simulink model "VissimConnector"  (R2021a)
settings: Solver=FixedStepDiscrete  StartTime=0.0  StopTime=Inf  RelTol=1e-3
libraries: drivingscenarioandsensors x2
settings Model: EnablePacing=on  PacingRate=0.200000  Creator=hichikaw  LastModifiedBy=itik
settings SolverCC: AlgebraicLoopSolver=TrustRegion
settings DataIOCC: SaveOutput=off  SignalLogging=off  DSMLogging=off  SaveTime=off  ReturnWorkspaceOutputs=off
settings OptimizationCC: DefaultParameterBehavior=Inlined  UseDivisionForNetSlopeComputation=on  GainParamInheritBuiltInType=on  UseFloatMulNetSlope=on  InlineInvariantSignals=on  PassReuseOutputArgsAs=Individual arguments  ZeroExternalMemoryAtStartup=off  ZeroInternalMemoryAtStartup=off  NoFixptDivByZeroProtection=on  EfficientFloat2IntCast=on  LifeSpan=1  OptimizeBlockOrder=speed  DifferentSizesBufferReuse=on  EfficientTunableParamExpr=on
settings DebuggingCC: ParameterTunabilityLossMsg=error  SFMachineParentedDataDiag=warning
settings HardwareCC: ProdLongLongMode=on
settings SFSimCC: MATLABDynamicMemAlloc=off
settings RTWCC: SystemTargetFile=ert.tlc  TemplateMakefile=ert_default_tmf
settings CodeAppCC: ForceParamTrailComments=on  IgnoreCustomStorageClasses=off  OperatorAnnotations=on  SimulinkDataObjDesc=on  SFDataObjDesc=on  CustomSymbolStrGlobalVar=rt$N$M  CustomSymbolStrType=$N$M  CustomSymbolStrFcn=$N$M$F  CustomSymbolStrMacro=$N$M  InsertBlockDesc=on
settings ERTTargetCC: TargetLangStandard=C99 (ISO)  GenerateSampleERTMain=on  IncludeMdlTerminateFcn=off  CombineSignalStateStructs=on  SuppressErrorStatus=on  SupportAbsoluteTime=off  SupportComplex=off  InlinedParameterPlacement=NonHierarchical  ERTCustomFileTemplate=example_file_process.tlc  ERTFilePackagingFormat=CompactWithDataFile

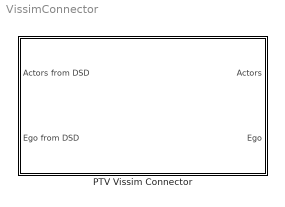
== system VissimConnector ==
  PTV Vissim Connector : Subsystem  mask{msk_strFilename=MyVIssimScenario.inpx, msk_dFrequency=10, msk_dRadius=-1, msk_dMaxNumActors=50, msk_strVissimConnectorDLLFile=./dll/VissimConnectorDLL.dll, msk_strInterfaceDLLFile=./dll/VissimInterfaceInterface.dll, msk_strVissimDLLFile=C:\Program Files\PTV Vision\PTV Vissim 2021\API\DrivingSimulator_DLL\bin\VS2013\x64\DrivingSimulatorProxy.dll}
      mask prompts: msk_strFilename "Vissim file name (*.inpx)"; msk_dFrequency "Vissim simulation frequency (Hz)"; msk_dRadius "Radius to detect actors (m)"; msk_dMaxNumActors "Maximum number of actors"; msk_strVissimConnectorDLLFile "Path to Vissim Connnector DLL<br/>(VissimConnectorDLL.dll)"; msk_strInterfaceDLLFile "Path to Vissim Interface DLL file<br/>(VissimInterfaceInterface.dll)"; msk_strVissimDLLFile "Path to Driving Simulator Proxy DLL<br/>(DrivingSimulatorProxy.dll)"
      mask DialogControl DescTextVar Prompt: Connect to PTV Vissim and interact traffic flow.
      mask DialogControl tab1 Prompt: Parameters
      mask DialogControl msk_btnSelectFile1 Prompt: Select file...
      mask DialogControl msk_btnSelectFile1 Callback:
      | filename = callbackFilenameFromDialog(...
      |     {...
      |         '*.inpx','Vissim (*.inpx)'
      |         '*.*','All (*.*)'}, ...
      |     gcb,'msk_strFilename');
      mask DialogControl Control6 Prompt: (Add text here)
      mask DialogControl tab2 Prompt: Configuration
      mask DialogControl msk_btnSelectFile2 Prompt: Select file...
      mask DialogControl msk_btnSelectFile2 Callback:
      | filename = callbackFilenameFromDialog(...
      |     {...
      |         '*.dll','DLL file (*.dll)'
      |         '*.*','All (*.*)'}, ...
      |     gcb,'msk_strVissimConnectorDLLFile');
      mask DialogControl msk_btnSelectFile3 Prompt: Select file...
      mask DialogControl msk_btnSelectFile3 Callback:
      | filename = callbackFilenameFromDialog(...
      |     {...
      |         '*.dll','DLL file (*.dll)'
      |         '*.*','All (*.*)'}, ...
      |     gcb,'msk_strInterfaceDLLFile');
      mask DialogControl msk_btnSelectFile4 Prompt: Select file...
      mask DialogControl msk_btnSelectFile4 Callback:
      | filename = callbackFilenameFromDialog(...
      |     {...
      |         '*.dll','DLL file (*.dll)'
      |         '*.*','All (*.*)'}, ...
      |     gcb,'msk_strVissimDLLFile');
      mask Display:
      | I=imread('PTVVissimLogo.png'); % Use "Edit Image" on toolstrip to change.
      | I=I/3+170;
      | image(I);

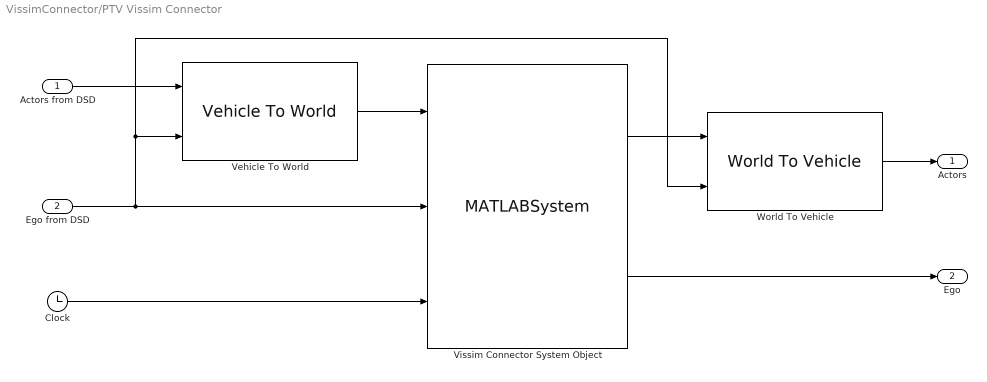
== system VissimConnector/PTV Vissim Connector ==
  Actors from DSD : Inport
  Ego from DSD : Inport  Port=2
  Clock : Clock
  Vehicle To World : drivingscenarioandsensors/Vehicle To World  BusNameSource=Auto  BusName=BusVehicleToWorldActors  SimulateUsing=Interpreted execution
      settings: SourceProductBaseCode=DR
  Vissim Connector System Object : MATLABSystem  System=VissimConnectorSO  m_strFilename=msk_strFilename  m_dFrequency=msk_dFrequency  m_dRadius=msk_dRadius  m_dMaxNumActors=msk_dMaxNumActors  m_strVissimConnectorDLLFile=./VissimConnectorDLL/x64/Release/VissimConnectorDLL.dll  m_strInterfaceDLLFile=./VissimInterface/VissimInterfaceInterface.dll  m_strVissimDLLFile=C:\Program Files\PTV Vision\PTV Vissim 2021\API\DrivingSimulator_DLL\bin\VS2013\x64\DrivingSimulatorProxy.dll  SimulateUsing=Interpreted execution
      mask Type: VissimConnectorSO
      mask Display:
      | disp('VissimConnectorSO');
      | port_label('input',1,'actorsIn');
      | port_label('input',2,'egoIn');
      | port_label('input',3,'simTime');
      | port_label('output',1,'actorsOut');
      | port_label('output',2,'egoOut');
  World To Vehicle : drivingscenarioandsensors/World To Vehicle  BusNameSource=Auto  BusName=BusWorldToVehicleActors  SimulateUsing=Interpreted execution
      settings: SourceProductBaseCode=DR
  Actors : Outport
  Ego : Outport  Port=2
  wires:
  Clock/1 -> Vissim Connector System Object/3
  Vissim Connector System Object/2 -> Ego/1
  Actors from DSD/1 -> Vehicle To World/1
  Ego from DSD/1 -> World To Vehicle/2, Vehicle To World/2, Vissim Connector System Object/2
  Vehicle To World/1 -> Vissim Connector System Object/1
  World To Vehicle/1 -> Actors/1
  Vissim Connector System Object/1 -> World To Vehicle/1
